simulink model "VascaNonLineareRealizazzioneIndustriale"  (R2022a)
settings: Solver=ode23s  StartTime=0.0  StopTime=6000  RelTol=1e-3
values from neighbouring files (symbols this model uses):
  Area = 0.08    [ControlloVasca.m]
  Au = 43*1e-6    (= 4.3e-05)    [ControlloVasca.m]
  bx = 0.1    [ControlloVasca.m]
  g = 9.8    [ControlloVasca.m]
  hu = -0.095    [ControlloVasca.m]
  KI = ((-153*0.0027)*abs(pole(G)))/0.007729    [ControlloVasca.m]
  KP = KI/abs(pole(G))    [ControlloVasca.m]
  L_T = 0:0.01:0.2    [ControlloVasca.m]
  mol1 = 0.07    [ControlloVasca.m]
  mol2 = 0.16    [ControlloVasca.m]
  Q_A = 1e-6*[0 8.8 24.6 42.0 57.1 72.4 86.1 102.3 117.6 132.0 144.9]    [ControlloVasca.m]
  rit1 = 2*tsign    (= 1000)    [ControlloVasca.m]
  rit2 = 4*tsign    (= 2000)    [ControlloVasca.m]
  Tn_A = 0:0.5:5    [ControlloVasca.m]
  Tn_T = [4.5221 4.4452 4.2412 3.9653 3.7932 3.5179 3.2742 3.0624 2.8349 2.5936 2.3522 2.1423 1.9151 1.6591 1.4251 1.1892 0.9053 0.7329 0.4750 0.2664 0.0471]    [ControlloVasca.m]
  tsign = 500    [ControlloVasca.m]
  y0 = 0.1    [ControlloVasca.m]
undefined symbols (not defined in the file or in its folder): bu
settings Model: LastModifiedBy=cl481357
settings OptimizationCC: BlockReduction=off  BooleanDataType=off
settings DebuggingCC: SaveWithParameterizedLinksMsg=none  UnderspecifiedInitializationDetection=Classic  MergeDetectMultiDrivingBlocksExec=none  SignalResolutionControl=TryResolveAllWithWarning
settings HardwareCC: TargetUnknown=on
settings ModelReferenceCC: PropagateSignalLabelsOutOfModel=off

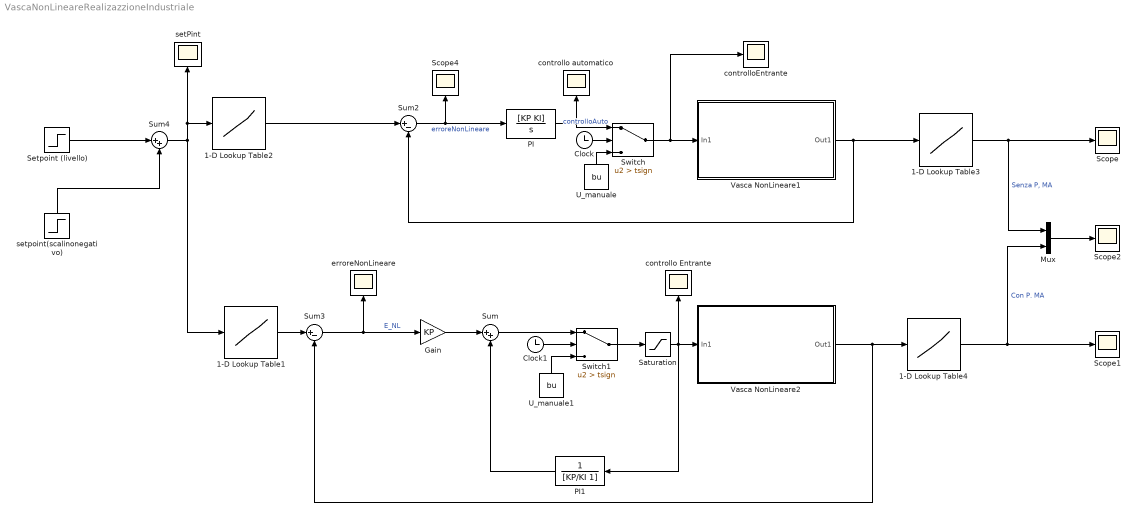
== system VascaNonLineareRealizazzioneIndustriale ==
  1-D Lookup Table1 : Lookup_n-D  NumberOfTableDimensions=1  BreakpointsForDimension1=L_T  Table=Tn_T  InternalRulePriority=Speed  RndMeth=Simplest
  1-D Lookup Table2 : Lookup_n-D  NumberOfTableDimensions=1  BreakpointsForDimension1=L_T  Table=Tn_T  InternalRulePriority=Speed  RndMeth=Simplest
  1-D Lookup Table3 : Lookup_n-D  NumberOfTableDimensions=1  BreakpointsForDimension1=fliplr(Tn_T)  Table=fliplr(L_T)  InternalRulePriority=Speed  RndMeth=Simplest
  1-D Lookup Table4 : Lookup_n-D  NumberOfTableDimensions=1  BreakpointsForDimension1=fliplr(Tn_T)  Table=fliplr(L_T)  InternalRulePriority=Speed  RndMeth=Simplest
  Clock : Clock
  Clock1 : Clock
  Gain : Gain  Gain=KP
  Mux : Mux  Inputs=2
  PI : TransferFcn  Numerator=[KP KI]  Denominator=[1 0]
  PI1 : TransferFcn  Denominator=[KP/KI 1]
  Saturation : Saturate  UpperLimit=5  LowerLimit=0
  Scope{,1..2,4} (4 alike) : Scope
  Setpoint (livello) : Step  Before=y0  After=y0+mol1  SampleTime=rit1  VectorParams1D=off
  Sum : Sum  Inputs=|++
  Sum2 : Sum  Inputs=|+-
  Sum3 : Sum  Inputs=|+-
  Sum4 : Sum  Inputs=|++
  Switch : Switch  Criteria=u2 > Threshold  Threshold=tsign  SaturateOnIntegerOverflow=off  InputSameDT=off
  Switch1 : Switch  Criteria=u2 > Threshold  Threshold=tsign  SaturateOnIntegerOverflow=off  InputSameDT=off
  U_manuale : Constant  Value=bu
  U_manuale1 : Constant  Value=bu
  Vasca NonLineare1 : Subsystem
  Vasca NonLineare2 : Subsystem
  controllo Entrante : Scope
  controllo automatico : Scope
  controlloEntrante : Scope
  erroreNonLineare : Scope
  setPint : Scope
  setpoint(scalinonegativo) : Step  After=-mol2  SampleTime=rit2  VectorParams1D=off  ZeroCross=off
  wires:
  Sum2/1 -> Scope4/1, PI/1  "erroreNonLineare"
  Sum3/1 -> Gain/1, erroreNonLineare/1  "E_NL"
  Vasca NonLineare2/1(Out1) -> 1-D Lookup Table4/1, Sum3/2
  1-D Lookup Table2/1 -> Sum2/1
  1-D Lookup Table1/1 -> Sum3/1
  1-D Lookup Table4/1 -> Mux/2, Scope1/1  "Con P. MA"
  Mux/1 -> Scope2/1
  Vasca NonLineare1/1(Out1) -> 1-D Lookup Table3/1, Sum2/2
  1-D Lookup Table3/1 -> Scope/1, Mux/1  "Senza P, MA"
  Setpoint (livello)/1 -> Sum4/1
  setpoint(scalinonegativo)/1 -> Sum4/2
  Sum4/1 -> 1-D Lookup Table1/1, 1-D Lookup Table2/1, setPint/1
  Clock/1 -> Switch/2
  PI/1 -> Switch/1, controllo automatico/1  "controlloAuto"
  Switch/1 -> controlloEntrante/1, Vasca NonLineare1/1(In1)
  Saturation/1 -> Vasca NonLineare2/1(In1), controllo Entrante/1, PI1/1
  Switch1/1 -> Saturation/1
  U_manuale1/1 -> Switch1/3
  Clock1/1 -> Switch1/2
  Gain/1 -> Sum/1
  PI1/1 -> Sum/2
  Sum/1 -> Switch1/1
  U_manuale/1 -> Switch/3

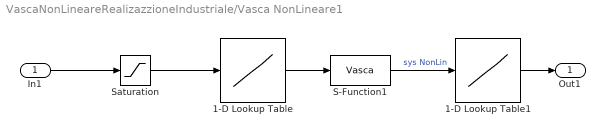
== system VascaNonLineareRealizazzioneIndustriale/Vasca NonLineare1 ==
  In1 : Inport
  1-D Lookup Table : Lookup_n-D  NumberOfTableDimensions=1  BreakpointsForDimension1=Tn_A  Table=Q_A  InternalRulePriority=Speed  RndMeth=Simplest
  1-D Lookup Table1 : Lookup_n-D  NumberOfTableDimensions=1  BreakpointsForDimension1=L_T  Table=Tn_T  InternalRulePriority=Speed  RndMeth=Simplest
  S-Function1 : S-Function  FunctionName=Vasca  Parameters=bx,Area,Au,g,hu  SFunctionDeploymentMode=off  EnableBusSupport=off
  Saturation : Saturate  UpperLimit=5  LowerLimit=0
  Out1 : Outport
  wires:
  S-Function1/1 -> 1-D Lookup Table1/1  "sys NonLin"
  1-D Lookup Table/1 -> S-Function1/1
  1-D Lookup Table1/1 -> Out1/1
  Saturation/1 -> 1-D Lookup Table/1
  In1/1 -> Saturation/1

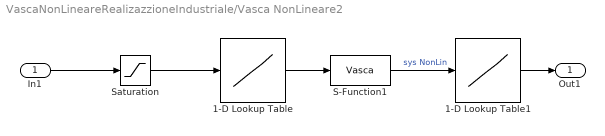
== system VascaNonLineareRealizazzioneIndustriale/Vasca NonLineare2 ==
  In1 : Inport
  1-D Lookup Table : Lookup_n-D  NumberOfTableDimensions=1  BreakpointsForDimension1=Tn_A  Table=Q_A  InternalRulePriority=Speed  RndMeth=Simplest
  1-D Lookup Table1 : Lookup_n-D  NumberOfTableDimensions=1  BreakpointsForDimension1=L_T  Table=Tn_T  InternalRulePriority=Speed  RndMeth=Simplest
  S-Function1 : S-Function  FunctionName=Vasca  Parameters=bx,Area,Au,g,hu  SFunctionDeploymentMode=off  EnableBusSupport=off
  Saturation : Saturate  UpperLimit=5  LowerLimit=0
  Out1 : Outport
  wires:
  S-Function1/1 -> 1-D Lookup Table1/1  "sys NonLin"
  1-D Lookup Table/1 -> S-Function1/1
  1-D Lookup Table1/1 -> Out1/1
  Saturation/1 -> 1-D Lookup Table/1
  In1/1 -> Saturation/1
